simulink model "drive_impl"  (R2021a)
settings: Solver=ode23s  StartTime=0.0  StopTime=5  FixedStep=1e-4  MaxStep=1e-3  RelTol=1e-3  EnableMultiTasking=on
InitFcn:
  | run('balancing_in_one_place_code.m');
values from neighbouring files (symbols this model uses):
  Cm = Ce    (= 0.0527)    [drive_params.m]
  h_val = R*2    (= 0.228)    [drive_imp_code.m]
  J_rolik = 1/4*m_rolik*r_val^2 + 1/12*m_rolik*h_val^2    [Initial_code.m]    (also in drive_imp_code.m = 4.5350625e-08)
  J_sphere = 2*M*R^2/5    (= 0.0038988)    [Initial_code.m]    (also in drive_imp_code.m)
  K_reg = place(A,B,p)    [Initial_code.m]    (also in drive_imp_code.m)
  Kconv = Udc    [drive_params.m]
  Kfb_i = 1/In    [drive_params.m]
  Ki = Te/(2*Kfb_i*(1/Cma)*Tconv*Kconv/Cea*b)    [drive_params.m]
  Klship = 1    [drive_params.m]
  L = 0.3    [Initial_code.m]    (also in drive_imp_code.m = 0.5)
  lenght_rolik = R+r_val    (= 0.1425)    [Initial_code.m]    (also in drive_imp_code.m)
  m = 1.5    [Initial_code.m]    (also in drive_imp_code.m)
  M = 0.75    [Initial_code.m]    (also in drive_imp_code.m)
  m_rolik = 1e-5    (= 1e-05)    [Initial_code.m]    (also in drive_imp_code.m)
  R = 0.114    [Initial_code.m]    (also in drive_imp_code.m)
  r_val = R*0.25    (= 0.0285)    [Initial_code.m]    (also in drive_imp_code.m)
  T = Tk    (= 1e-05)    [drive_params.m]
  Tconv = 0.5*T    (= 5e-06)    [drive_params.m]
  Ti = Te    (= 0.000136363636364)    [drive_params.m]
  U_nom = 12    [drive_params.m]
undefined symbols (not defined in the file or in its folder): DiscIntNeverNeededParam, X, Y, Z
libraries: sm_lib x87, nesl_utility x32, fl_lib x23, simulink x10, fl_ps_legacy_lib x9, ee_lib x8, simulink_extras x4, pid_lib x1
(part 4 of 4)

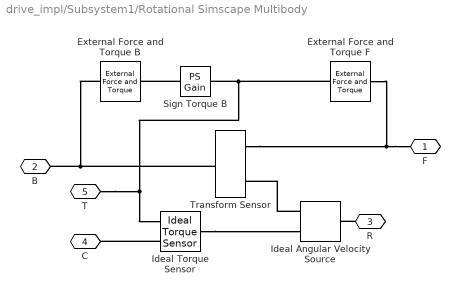
== system drive_impl/Subsystem1/Rotational Simscape Multibody ==
  External Force and Torque B : sm_lib/Forces and Torques/External Force and Torque  ForceResolutionFrame=AttachedFrame  EnableForceX=off  EnableForceY=off  EnableForceZ=off  EnableForce=off  TorqueResolutionFrame=AttachedFrame  EnableTorqueX=off  EnableTorqueY=off  EnableTorqueZ=on  EnableTorque=off
  External Force and Torque F : sm_lib/Forces and Torques/External Force and Torque  ForceResolutionFrame=AttachedFrame  EnableForceX=off  EnableForceY=off  EnableForceZ=off  EnableForce=off  TorqueResolutionFrame=AttachedFrame  EnableTorqueX=off  EnableTorqueY=off  EnableTorqueZ=on  EnableTorque=off
  Ideal Angular Velocity Source : fl_lib/Mechanical/Mechanical Sources/Ideal Angular Velocity Source
  Ideal Torque Sensor : fl_lib/Mechanical/Mechanical Sensors/Ideal Torque Sensor
  Sign Torque B : fl_ps_legacy_lib/Legacy Physical Signals/Functions/PS Gain  gain=-1
  Transform Sensor : sm_lib/Frames and Transforms/Transform Sensor  MeasurementFrame=Base  SenseAngle=off  SenseAxis=off  SenseAngle1=off  SenseAngle2=off  SenseAngle3=off  SenseQ=off  SenseR=off  SenseOmegaX=off  SenseOmegaY=off  SenseOmegaZ=on  SenseOmega1=off  SenseOmega2=off  SenseOmega3=off  SenseQDot=off  SenseRDot=off  SenseAlphaX=off  SenseAlphaY=off  SenseAlphaZ=off  SenseAlpha1=off  SenseAlpha2=off  SenseAlpha3=off  SenseQDDot=off  SenseRDDot=off  SenseX=off  SenseY=off  SenseZ=off  SenseRad=off  SenseAzim=off  SenseDist=off  SenseInc=off  SenseXDot=off  SenseYDot=off  SenseZDot=off  SenseRadDot=off  SenseAzimDot=off  SenseDistDot=off  SenseIncDot=off  SenseXDDot=off  SenseYDDot=off  SenseZDDot=off  SenseRadDDot=off  SenseAzimDDot=off  SenseDistDDot=off  SenseIncDDot=off
  F : PMIOPort  Side=Right
  B : PMIOPort  Port=2  Side=Left
  R : PMIOPort  Port=3  Side=Right
  C : PMIOPort  Port=4  Side=Left
  T : PMIOPort  Port=5  Side=Right
  connections:
  Sign Torque B/LConn1 -- T/RConn1 -- Ideal Torque Sensor/RConn2 -- External Force and Torque F/LConn1
  Sign Torque B/RConn1 -- External Force and Torque B/LConn1
  Ideal Angular Velocity Source/RConn1 -- Transform Sensor/RConn2
  F/RConn1 -- External Force and Torque F/RConn1 -- Transform Sensor/RConn1
  External Force and Torque B/RConn1 -- B/RConn1 -- Transform Sensor/LConn1
  Ideal Torque Sensor/LConn1 -- Ideal Angular Velocity Source/RConn2
  R/RConn1 -- Ideal Angular Velocity Source/LConn1
  Ideal Torque Sensor/RConn1 -- C/RConn1

== system drive_impl/Subsystem1/Subsystem1 ==
  Brick Solid : sm_lib/Body Elements/Brick Solid  GraphicAmbientColor=[0.15 0.15 0.15 1.0]  BasedOnType=Mass  BrickDimensions=[2*RolikRadius RolikLenght RolikRadius/10]  BrickDimensionUnits=m  CenterOfMass=[0 0 0]  CenterOfMassUnits=m  GraphicDiffuseColor=[1.0 0.2 0.2]  Density=1000  DensityUnits=kg/m^3  DoExposeReferenceFrame=on  GraphicEmissiveColor=[0.0 0.0 0.0 1.0]  ExportEntireGeometry=off  SerializedFrames=<Frames/>  MarkerShape=Sphere  MarkerSize=10  GraphicType=FromGeometry  InertiaType=CalculateFromGeometry  Mass=1e-6  MassUnits=kg  MomentsOfInertia=[1 1 1]  MomentsOfInertiaUnits=kg*m^2  GraphicOpacity=0.5  ProductsOfInertia=[0 0 0]  ProductsOfInertiaUnits=kg*m^2  GraphicShininess=75  GraphicSpecularColor=[0.5 0.5 0.5 1.0]  GraphicVisPropType=SimpleVisualProperties
  Brick Solid1 : sm_lib/Body Elements/Brick Solid  GraphicAmbientColor=[0.15 0.15 0.15 1.0]  BasedOnType=Mass  BrickDimensions=[2*RolikRadius RolikLenght RolikRadius/10]  BrickDimensionUnits=m  CenterOfMass=[0 0 0]  CenterOfMassUnits=m  GraphicDiffuseColor=[1.0 0.2 0.2]  Density=1000  DensityUnits=kg/m^3  DoExposeReferenceFrame=on  GraphicEmissiveColor=[0.0 0.0 0.0 1.0]  ExportEntireGeometry=off  SerializedFrames=<Frames/>  MarkerShape=Sphere  MarkerSize=10  GraphicType=FromGeometry  InertiaType=CalculateFromGeometry  Mass=1e-6  MassUnits=kg  MomentsOfInertia=[1 1 1]  MomentsOfInertiaUnits=kg*m^2  GraphicOpacity=0.5  ProductsOfInertia=[0 0 0]  ProductsOfInertiaUnits=kg*m^2  GraphicShininess=75  GraphicSpecularColor=[0.5 0.5 0.5 1.0]  GraphicVisPropType=SimpleVisualProperties
  Cylindrical Solid26 : sm_lib/Body Elements/Cylindrical Solid  GraphicAmbientColor=[0.15 0.15 0.15 1.0]  BasedOnType=Mass  CenterOfMass=[0 0 0]  CenterOfMassUnits=m  GraphicDiffuseColor=[0.2 1.0 0.2]  CylinderLength=RolikLenght  CylinderLengthUnits=m  CylinderRadius=RolikRadius  CylinderRadiusUnits=m  Density=1000  DensityUnits=kg/m^3  DoExposeReferenceFrame=on  GraphicEmissiveColor=[0.0 0.0 0.0 1.0]  ExportEntireGeometry=off  SerializedFrames=<Frames/>  MarkerShape=Sphere  MarkerSize=10  GraphicType=FromGeometry  InertiaType=CalculateFromGeometry  Mass=m_rolik  MassUnits=kg  MomentsOfInertia=[1 1 1]  MomentsOfInertiaUnits=kg*m^2  GraphicOpacity=0.6  ProductsOfInertia=[0 0 0]  ProductsOfInertiaUnits=kg*m^2  GraphicShininess=75  GraphicSpecularColor=[0.5 0.5 0.5 1.0]  GraphicVisPropType=SimpleVisualProperties
  Rigid Transform7 : sm_lib/Frames and Transforms/Rigid Transform  TranslationMethod=None  TranslationStandardOffset=0  TranslationLengthUnit=m  TranslationStandardAxis=+Z  TranslationCartesianOffset=[0 0 0]  TranslationROffset=0  TranslationROffsetUnits=m  TranslationZOffset=0  TranslationZOffsetUnits=m  TranslationThetaOffset=0  TranslationThetaOffsetUnits=deg  RotationMethod=StandardAxis  RotationAngleUnits=deg  RotationStandardAxis=+X  RotationAngle=90  RotationArbitraryAxis=[0 0 1]  FollAlignAxisA=+X  BaseAlignAxisA=+Y  FollAlignAxisB=+Y  BaseAlignAxisB=+Z  RotationSequenceAxes=FollowerAxes  RotationSequence=XYX  RotationSequenceAngles=[0 0 0]  RotationSequenceAnglesUnits=deg  RotationMatrix=[1 0 0; 0 1 0; 0 0 1]
  Rigid Transform8 : sm_lib/Frames and Transforms/Rigid Transform  TranslationMethod=None  TranslationStandardOffset=0  TranslationLengthUnit=m  TranslationStandardAxis=+Z  TranslationCartesianOffset=[0 0 0]  TranslationROffset=0  TranslationROffsetUnits=m  TranslationZOffset=0  TranslationZOffsetUnits=m  TranslationThetaOffset=0  TranslationThetaOffsetUnits=deg  RotationMethod=StandardAxis  RotationAngleUnits=deg  RotationStandardAxis=+Y  RotationAngle=90  RotationArbitraryAxis=[0 0 1]  FollAlignAxisA=+X  BaseAlignAxisA=+Y  FollAlignAxisB=+Y  BaseAlignAxisB=+Z  RotationSequenceAxes=FollowerAxes  RotationSequence=XYX  RotationSequenceAngles=[0 0 0]  RotationSequenceAnglesUnits=deg  RotationMatrix=[1 0 0; 0 1 0; 0 0 1]
  Conn1 : PMIOPort  Side=Left
  connections:
  Cylindrical Solid26/RConn1 -- Rigid Transform7/LConn1 -- Conn1/RConn1
  Brick Solid1/RConn1 -- Rigid Transform8/RConn1
  Brick Solid/RConn1 -- Rigid Transform7/RConn1 -- Rigid Transform8/LConn1

== system drive_impl/Subsystem1/Основание4 ==
  Rigid Transform : sm_lib/Frames and Transforms/Rigid Transform  TranslationMethod=None  TranslationStandardOffset=0  TranslationLengthUnit=m  TranslationStandardAxis=+Z  TranslationCartesianOffset=[0 0 0]  TranslationROffset=0  TranslationROffsetUnits=m  TranslationZOffset=0  TranslationZOffsetUnits=m  TranslationThetaOffset=0  TranslationThetaOffsetUnits=deg  RotationMethod=StandardAxis  RotationAngleUnits=deg  RotationStandardAxis=+X  RotationAngle=90  RotationArbitraryAxis=[0 0 1]  FollAlignAxisA=+X  BaseAlignAxisA=+Y  FollAlignAxisB=+Y  BaseAlignAxisB=+Z  RotationSequenceAxes=FollowerAxes  RotationSequence=XYX  RotationSequenceAngles=[0 0 0]  RotationSequenceAnglesUnits=deg  RotationMatrix=[1 0 0; 0 1 0; 0 0 1]
  Rigid Transform1 : sm_lib/Frames and Transforms/Rigid Transform  TranslationMethod=None  TranslationStandardOffset=0  TranslationLengthUnit=m  TranslationStandardAxis=+Z  TranslationCartesianOffset=[0 0 0]  TranslationROffset=0  TranslationROffsetUnits=m  TranslationZOffset=0  TranslationZOffsetUnits=m  TranslationThetaOffset=0  TranslationThetaOffsetUnits=deg  RotationMethod=StandardAxis  RotationAngleUnits=deg  RotationStandardAxis=+Y  RotationAngle=90  RotationArbitraryAxis=[0 0 1]  FollAlignAxisA=+X  BaseAlignAxisA=+Y  FollAlignAxisB=+Y  BaseAlignAxisB=+Z  RotationSequenceAxes=FollowerAxes  RotationSequence=XYX  RotationSequenceAngles=[0 0 0]  RotationSequenceAnglesUnits=deg  RotationMatrix=[1 0 0; 0 1 0; 0 0 1]
  Solid1 : sm_lib/Body Elements/Spherical Solid  GraphicAmbientColor=[0.15 0.15 0.15 1.0]  BasedOnType=Mass  CenterOfMass=[0 0 0]  CenterOfMassUnits=m  GraphicDiffuseColor=[1.0 1.0 0.0]  Density=1000  DensityUnits=kg/m^3  DoExposeReferenceFrame=on  GraphicEmissiveColor=[0.0 0.0 0.0 1.0]  ExportEntireGeometry=off  SerializedExposedGeometries=<ExposedGeometries/>  SerializedFrames=<Frames/>  MarkerShape=Sphere  MarkerSize=10  GraphicType=FromGeometry  InertiaType=CalculateFromGeometry  Mass=Mass  MassUnits=kg  MomentsOfInertia=[1 1 1]  MomentsOfInertiaUnits=kg*m^2  GraphicOpacity=1.0  ProductsOfInertia=[1 1 1]  ProductsOfInertiaUnits=kg*m^2  GraphicShininess=75  GraphicSpecularColor=[0.5 0.5 0.5 1.0]  SphereRadius=SphereRadius  SphereRadiusUnits=m  GraphicVisPropType=SimpleVisualProperties
  Solid2 : sm_lib/Body Elements/Revolved Solid  GraphicAmbientColor=[0.15 0.15 0.15 1.0]  BasedOnType=Mass  CenterOfMass=[0 0 0]  CenterOfMassUnits=m  GraphicDiffuseColor=[1.0 0.0 0.0]  ExportConvexHullGeometry=off  Density=1000  DensityUnits=kg/m^3  DoExposeReferenceFrame=on  GraphicEmissiveColor=[0.0 0.0 0.0 1.0]  ExportEntireGeometry=off  SerializedFrames=<Frames/>  MarkerShape=Sphere  MarkerSize=10  GraphicType=FromGeometry  InertiaType=CalculateFromGeometry  Mass=0  MassUnits=kg  MomentsOfInertia=[1 1 1]  MomentsOfInertiaUnits=kg*m^2  GraphicOpacity=0.5  ProductsOfInertia=[1 1 1]  ProductsOfInertiaUnits=kg*m^2  RevolutionCrossSection=[0 SphereRadius*perc1; 0 -SphereRadius*perc1; SphereRadius*1.01 -SphereRadius*perc1; SphereRadius*1.01 SphereRadius*perc1]  RevolutionCrossSectionUnits=m  RevolutionAngle=180  RevolutionAngleUnits=deg  RevolutionExtent=Full  GraphicShininess=75  GraphicSpecularColor=[0.5 0.5 0.5 1.0]  GraphicVisPropType=SimpleVisualProperties
  Solid3 : sm_lib/Body Elements/Revolved Solid  GraphicAmbientColor=[0.15 0.15 0.15 1.0]  BasedOnType=Mass  CenterOfMass=[0 0 0]  CenterOfMassUnits=m  GraphicDiffuseColor=[1.0 0.0 0.0]  ExportConvexHullGeometry=off  Density=1000  DensityUnits=kg/m^3  DoExposeReferenceFrame=on  GraphicEmissiveColor=[0.0 0.0 0.0 1.0]  ExportEntireGeometry=off  SerializedFrames=<Frames/>  MarkerShape=Sphere  MarkerSize=10  GraphicType=FromGeometry  InertiaType=CalculateFromGeometry  Mass=0  MassUnits=kg  MomentsOfInertia=[1 1 1]  MomentsOfInertiaUnits=kg*m^2  GraphicOpacity=0.5  ProductsOfInertia=[1 1 1]  ProductsOfInertiaUnits=kg*m^2  RevolutionCrossSection=[0 SphereRadius*perc1; 0 -SphereRadius*perc1; SphereRadius*perc2 -SphereRadius*perc1; SphereRadius*perc2 SphereRadius*perc1]  RevolutionCrossSectionUnits=m  RevolutionAngle=180  RevolutionAngleUnits=deg  RevolutionExtent=Full  GraphicShininess=75  GraphicSpecularColor=[0.5 0.5 0.5 1.0]  GraphicVisPropType=SimpleVisualProperties
  Solid4 : sm_lib/Body Elements/Revolved Solid  GraphicAmbientColor=[0.15 0.15 0.15 1.0]  BasedOnType=Mass  CenterOfMass=[0 0 0]  CenterOfMassUnits=m  GraphicDiffuseColor=[1.0 0.0 0.0]  ExportConvexHullGeometry=off  Density=1000  DensityUnits=kg/m^3  DoExposeReferenceFrame=on  GraphicEmissiveColor=[0.0 0.0 0.0 1.0]  ExportEntireGeometry=off  SerializedFrames=<Frames/>  MarkerShape=Sphere  MarkerSize=10  GraphicType=FromGeometry  InertiaType=CalculateFromGeometry  Mass=0  MassUnits=kg  MomentsOfInertia=[1 1 1]  MomentsOfInertiaUnits=kg*m^2  GraphicOpacity=0.5  ProductsOfInertia=[1 1 1]  ProductsOfInertiaUnits=kg*m^2  RevolutionCrossSection=[0 SphereRadius*perc1; 0 -SphereRadius*perc1; SphereRadius*perc2 -SphereRadius*perc1; SphereRadius*perc2 SphereRadius*perc1]  RevolutionCrossSectionUnits=m  RevolutionAngle=180  RevolutionAngleUnits=deg  RevolutionExtent=Full  GraphicShininess=75  GraphicSpecularColor=[0.5 0.5 0.5 1.0]  GraphicVisPropType=SimpleVisualProperties
  Conn1 : PMIOPort  Side=Left
  connections:
  Rigid Transform/LConn1 -- Solid2/RConn1 -- Solid1/RConn1 -- Conn1/RConn1
  Solid4/RConn1 -- Rigid Transform1/RConn1
  Rigid Transform1/LConn1 -- Rigid Transform/RConn1 -- Solid3/RConn1

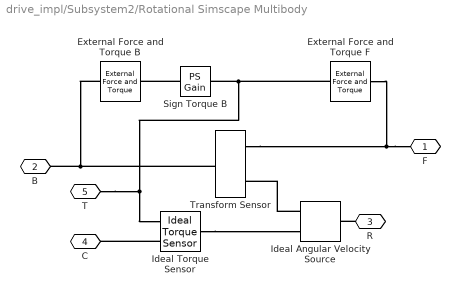
== system drive_impl/Subsystem2/Rotational Simscape Multibody ==
  External Force and Torque B : sm_lib/Forces and Torques/External Force and Torque  ForceResolutionFrame=AttachedFrame  EnableForceX=off  EnableForceY=off  EnableForceZ=off  EnableForce=off  TorqueResolutionFrame=AttachedFrame  EnableTorqueX=off  EnableTorqueY=off  EnableTorqueZ=on  EnableTorque=off
  External Force and Torque F : sm_lib/Forces and Torques/External Force and Torque  ForceResolutionFrame=AttachedFrame  EnableForceX=off  EnableForceY=off  EnableForceZ=off  EnableForce=off  TorqueResolutionFrame=AttachedFrame  EnableTorqueX=off  EnableTorqueY=off  EnableTorqueZ=on  EnableTorque=off
  Ideal Angular Velocity Source : fl_lib/Mechanical/Mechanical Sources/Ideal Angular Velocity Source
  Ideal Torque Sensor : fl_lib/Mechanical/Mechanical Sensors/Ideal Torque Sensor
  Sign Torque B : fl_ps_legacy_lib/Legacy Physical Signals/Functions/PS Gain  gain=-1
  Transform Sensor : sm_lib/Frames and Transforms/Transform Sensor  MeasurementFrame=Base  SenseAngle=off  SenseAxis=off  SenseAngle1=off  SenseAngle2=off  SenseAngle3=off  SenseQ=off  SenseR=off  SenseOmegaX=off  SenseOmegaY=off  SenseOmegaZ=on  SenseOmega1=off  SenseOmega2=off  SenseOmega3=off  SenseQDot=off  SenseRDot=off  SenseAlphaX=off  SenseAlphaY=off  SenseAlphaZ=off  SenseAlpha1=off  SenseAlpha2=off  SenseAlpha3=off  SenseQDDot=off  SenseRDDot=off  SenseX=off  SenseY=off  SenseZ=off  SenseRad=off  SenseAzim=off  SenseDist=off  SenseInc=off  SenseXDot=off  SenseYDot=off  SenseZDot=off  SenseRadDot=off  SenseAzimDot=off  SenseDistDot=off  SenseIncDot=off  SenseXDDot=off  SenseYDDot=off  SenseZDDot=off  SenseRadDDot=off  SenseAzimDDot=off  SenseDistDDot=off  SenseIncDDot=off
  F : PMIOPort  Side=Right
  B : PMIOPort  Port=2  Side=Left
  R : PMIOPort  Port=3  Side=Right
  C : PMIOPort  Port=4  Side=Left
  T : PMIOPort  Port=5  Side=Right
  connections:
  Sign Torque B/LConn1 -- T/RConn1 -- Ideal Torque Sensor/RConn2 -- External Force and Torque F/LConn1
  Sign Torque B/RConn1 -- External Force and Torque B/LConn1
  Ideal Angular Velocity Source/RConn1 -- Transform Sensor/RConn2
  F/RConn1 -- External Force and Torque F/RConn1 -- Transform Sensor/RConn1
  External Force and Torque B/RConn1 -- B/RConn1 -- Transform Sensor/LConn1
  Ideal Torque Sensor/LConn1 -- Ideal Angular Velocity Source/RConn2
  R/RConn1 -- Ideal Angular Velocity Source/LConn1
  Ideal Torque Sensor/RConn1 -- C/RConn1

== system drive_impl/Subsystem2/Основание4 ==
  Rigid Transform : sm_lib/Frames and Transforms/Rigid Transform  TranslationMethod=None  TranslationStandardOffset=0  TranslationLengthUnit=m  TranslationStandardAxis=+Z  TranslationCartesianOffset=[0 0 0]  TranslationROffset=0  TranslationROffsetUnits=m  TranslationZOffset=0  TranslationZOffsetUnits=m  TranslationThetaOffset=0  TranslationThetaOffsetUnits=deg  RotationMethod=StandardAxis  RotationAngleUnits=deg  RotationStandardAxis=+X  RotationAngle=90  RotationArbitraryAxis=[0 0 1]  FollAlignAxisA=+X  BaseAlignAxisA=+Y  FollAlignAxisB=+Y  BaseAlignAxisB=+Z  RotationSequenceAxes=FollowerAxes  RotationSequence=XYX  RotationSequenceAngles=[0 0 0]  RotationSequenceAnglesUnits=deg  RotationMatrix=[1 0 0; 0 1 0; 0 0 1]
  Rigid Transform1 : sm_lib/Frames and Transforms/Rigid Transform  TranslationMethod=None  TranslationStandardOffset=0  TranslationLengthUnit=m  TranslationStandardAxis=+Z  TranslationCartesianOffset=[0 0 0]  TranslationROffset=0  TranslationROffsetUnits=m  TranslationZOffset=0  TranslationZOffsetUnits=m  TranslationThetaOffset=0  TranslationThetaOffsetUnits=deg  RotationMethod=StandardAxis  RotationAngleUnits=deg  RotationStandardAxis=+Y  RotationAngle=90  RotationArbitraryAxis=[0 0 1]  FollAlignAxisA=+X  BaseAlignAxisA=+Y  FollAlignAxisB=+Y  BaseAlignAxisB=+Z  RotationSequenceAxes=FollowerAxes  RotationSequence=XYX  RotationSequenceAngles=[0 0 0]  RotationSequenceAnglesUnits=deg  RotationMatrix=[1 0 0; 0 1 0; 0 0 1]
  Solid1 : sm_lib/Body Elements/Spherical Solid  GraphicAmbientColor=[0.15 0.15 0.15 1.0]  BasedOnType=Mass  CenterOfMass=[0 0 0]  CenterOfMassUnits=m  GraphicDiffuseColor=[1.0 1.0 0.0]  Density=1000  DensityUnits=kg/m^3  DoExposeReferenceFrame=on  GraphicEmissiveColor=[0.0 0.0 0.0 1.0]  ExportEntireGeometry=off  SerializedExposedGeometries=<ExposedGeometries/>  SerializedFrames=<Frames/>  MarkerShape=Sphere  MarkerSize=10  GraphicType=FromGeometry  InertiaType=CalculateFromGeometry  Mass=Mass  MassUnits=kg  MomentsOfInertia=[1 1 1]  MomentsOfInertiaUnits=kg*m^2  GraphicOpacity=1.0  ProductsOfInertia=[1 1 1]  ProductsOfInertiaUnits=kg*m^2  GraphicShininess=75  GraphicSpecularColor=[0.5 0.5 0.5 1.0]  SphereRadius=SphereRadius  SphereRadiusUnits=m  GraphicVisPropType=SimpleVisualProperties
  Solid2 : sm_lib/Body Elements/Revolved Solid  GraphicAmbientColor=[0.15 0.15 0.15 1.0]  BasedOnType=Mass  CenterOfMass=[0 0 0]  CenterOfMassUnits=m  GraphicDiffuseColor=[1.0 0.0 0.0]  ExportConvexHullGeometry=off  Density=1000  DensityUnits=kg/m^3  DoExposeReferenceFrame=on  GraphicEmissiveColor=[0.0 0.0 0.0 1.0]  ExportEntireGeometry=off  SerializedFrames=<Frames/>  MarkerShape=Sphere  MarkerSize=10  GraphicType=FromGeometry  InertiaType=CalculateFromGeometry  Mass=0  MassUnits=kg  MomentsOfInertia=[1 1 1]  MomentsOfInertiaUnits=kg*m^2  GraphicOpacity=0.5  ProductsOfInertia=[1 1 1]  ProductsOfInertiaUnits=kg*m^2  RevolutionCrossSection=[0 SphereRadius*perc1; 0 -SphereRadius*perc1; SphereRadius*1.01 -SphereRadius*perc1; SphereRadius*1.01 SphereRadius*perc1]  RevolutionCrossSectionUnits=m  RevolutionAngle=180  RevolutionAngleUnits=deg  RevolutionExtent=Full  GraphicShininess=75  GraphicSpecularColor=[0.5 0.5 0.5 1.0]  GraphicVisPropType=SimpleVisualProperties
  Solid3 : sm_lib/Body Elements/Revolved Solid  GraphicAmbientColor=[0.15 0.15 0.15 1.0]  BasedOnType=Mass  CenterOfMass=[0 0 0]  CenterOfMassUnits=m  GraphicDiffuseColor=[1.0 0.0 0.0]  ExportConvexHullGeometry=off  Density=1000  DensityUnits=kg/m^3  DoExposeReferenceFrame=on  GraphicEmissiveColor=[0.0 0.0 0.0 1.0]  ExportEntireGeometry=off  SerializedFrames=<Frames/>  MarkerShape=Sphere  MarkerSize=10  GraphicType=FromGeometry  InertiaType=CalculateFromGeometry  Mass=0  MassUnits=kg  MomentsOfInertia=[1 1 1]  MomentsOfInertiaUnits=kg*m^2  GraphicOpacity=0.5  ProductsOfInertia=[1 1 1]  ProductsOfInertiaUnits=kg*m^2  RevolutionCrossSection=[0 SphereRadius*perc1; 0 -SphereRadius*perc1; SphereRadius*perc2 -SphereRadius*perc1; SphereRadius*perc2 SphereRadius*perc1]  RevolutionCrossSectionUnits=m  RevolutionAngle=180  RevolutionAngleUnits=deg  RevolutionExtent=Full  GraphicShininess=75  GraphicSpecularColor=[0.5 0.5 0.5 1.0]  GraphicVisPropType=SimpleVisualProperties
  Solid4 : sm_lib/Body Elements/Revolved Solid  GraphicAmbientColor=[0.15 0.15 0.15 1.0]  BasedOnType=Mass  CenterOfMass=[0 0 0]  CenterOfMassUnits=m  GraphicDiffuseColor=[1.0 0.0 0.0]  ExportConvexHullGeometry=off  Density=1000  DensityUnits=kg/m^3  DoExposeReferenceFrame=on  GraphicEmissiveColor=[0.0 0.0 0.0 1.0]  ExportEntireGeometry=off  SerializedFrames=<Frames/>  MarkerShape=Sphere  MarkerSize=10  GraphicType=FromGeometry  InertiaType=CalculateFromGeometry  Mass=0  MassUnits=kg  MomentsOfInertia=[1 1 1]  MomentsOfInertiaUnits=kg*m^2  GraphicOpacity=0.5  ProductsOfInertia=[1 1 1]  ProductsOfInertiaUnits=kg*m^2  RevolutionCrossSection=[0 SphereRadius*perc1; 0 -SphereRadius*perc1; SphereRadius*perc2 -SphereRadius*perc1; SphereRadius*perc2 SphereRadius*perc1]  RevolutionCrossSectionUnits=m  RevolutionAngle=180  RevolutionAngleUnits=deg  RevolutionExtent=Full  GraphicShininess=75  GraphicSpecularColor=[0.5 0.5 0.5 1.0]  GraphicVisPropType=SimpleVisualProperties
  Conn1 : PMIOPort  Side=Left
  connections:
  Rigid Transform/LConn1 -- Solid2/RConn1 -- Solid1/RConn1 -- Conn1/RConn1
  Solid4/RConn1 -- Rigid Transform1/RConn1
  Rigid Transform1/LConn1 -- Rigid Transform/RConn1 -- Solid3/RConn1

== system drive_impl/Subsystem3/DC Current Sensor ==
  Current Sensor : fl_lib/Electrical/Electrical Sensors/Current Sensor
      settings: LogSimulationData=on
  PS-Simulink Converter : nesl_utility/PS-Simulink Converter  PhysicalDomain=network_engine_domain  SubClassName=ps_output  LeftPortType=input  RightPortType=output  PseudoPeriodic=off  Frequencies=[]  Unit=1  AffineConversion=off
      settings: SourceProductBaseCode=PW,SS
  - : PMIOPort  Side=Left
  + : PMIOPort  Port=2  Side=Right
  tag scope: i_dc=global
  wires:
  PS-Simulink Converter/1 -> [i_dc]
  connections:
  Current Sensor/RConn2 -- -/RConn1
  +/RConn1 -- Current Sensor/LConn1
  Current Sensor/RConn1 -- PS-Simulink Converter/LConn1

== system drive_impl/Subsystem3/DC Voltage Sensor ==
  PS-Simulink Converter : nesl_utility/PS-Simulink Converter  PhysicalDomain=network_engine_domain  SubClassName=ps_output  LeftPortType=input  RightPortType=output  PseudoPeriodic=off  Frequencies=[]  Unit=1  AffineConversion=off
      settings: SourceProductBaseCode=PW,SS
  Voltage Sensor : fl_lib/Electrical/Electrical Sensors/Voltage Sensor
      settings: LogSimulationData=on
  - : PMIOPort  Side=Left
  + : PMIOPort  Port=2  Side=Right
  tag scope: v_dc=global
  wires:
  PS-Simulink Converter/1 -> [v_dc]
  connections:
  Voltage Sensor/LConn1 -- +/RConn1
  Voltage Sensor/RConn1 -- PS-Simulink Converter/LConn1
  Voltage Sensor/RConn2 -- -/RConn1

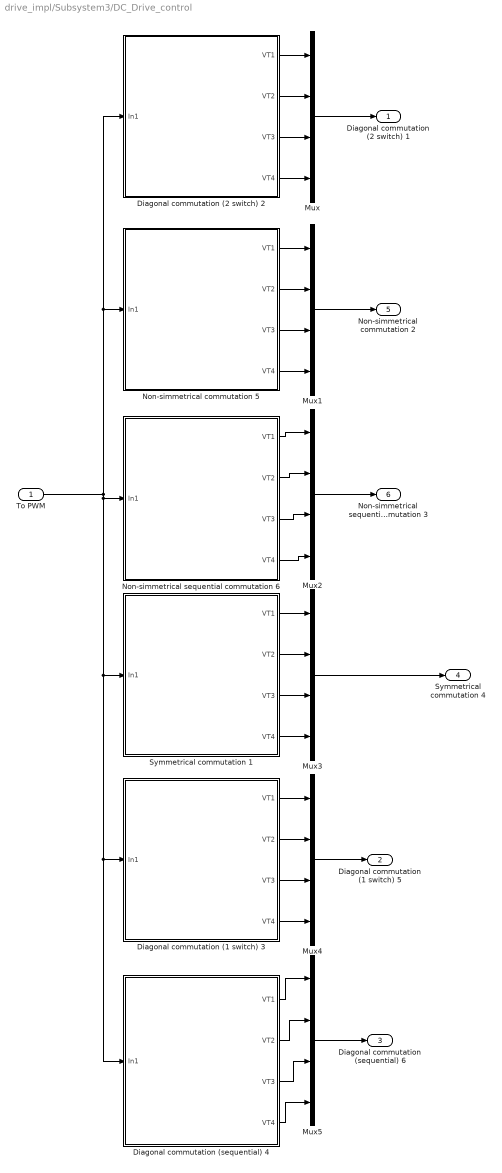
== system drive_impl/Subsystem3/DC_Drive_control ==
  To PWM : Inport
  Diagonal commutation (1 switch) 3 : Subsystem
  Diagonal commutation (2 switch) 2 : Subsystem
  Diagonal commutation (sequential) 4 : Subsystem
  Mux{,1..5} (6 alike) : Mux
  Non-simmetrical commutation 5 : Subsystem
  "Non-simmetrical sequential commutation 6 " : Subsystem
  Symmetrical commutation 1 : Subsystem
  Diagonal commutation (2 switch) 1 : Outport  VectorParamsAs1DForOutWhenUnconnected=off
  Diagonal commutation (1 switch) 5 : Outport  Port=2  VectorParamsAs1DForOutWhenUnconnected=off
  Diagonal commutation (sequential) 6 : Outport  Port=3  VectorParamsAs1DForOutWhenUnconnected=off
  Symmetrical commutation 4 : Outport  Port=4  VectorParamsAs1DForOutWhenUnconnected=off
  Non-simmetrical commutation 2 : Outport  Port=5  VectorParamsAs1DForOutWhenUnconnected=off
  "Non-simmetrical sequential commutation 3 " : Outport  Port=6  VectorParamsAs1DForOutWhenUnconnected=off
  wires:
  To PWM/1 -> "Non-simmetrical sequential commutation 6 "/1(In1), Diagonal commutation (1 switch) 3/1(In1), Diagonal commutation (sequential) 4/1(In1), Symmetrical commutation 1/1(In1), Diagonal commutation (2 switch) 2/1(In1), Non-simmetrical commutation 5/1(In1)
  Diagonal commutation (2 switch) 2/1(VT1) -> Mux/1
  Diagonal commutation (2 switch) 2/2(VT2) -> Mux/2
  Diagonal commutation (2 switch) 2/3(VT3) -> Mux/3
  Diagonal commutation (2 switch) 2/4(VT4) -> Mux/4
  Non-simmetrical commutation 5/1(VT1) -> Mux1/1
  Non-simmetrical commutation 5/2(VT2) -> Mux1/2
  Non-simmetrical commutation 5/3(VT3) -> Mux1/3
  Non-simmetrical commutation 5/4(VT4) -> Mux1/4
  "Non-simmetrical sequential commutation 6 "/3(VT3) -> Mux2/3
  "Non-simmetrical sequential commutation 6 "/4(VT4) -> Mux2/4
  "Non-simmetrical sequential commutation 6 "/2(VT2) -> Mux2/2
  Symmetrical commutation 1/4(VT4) -> Mux3/4
  Symmetrical commutation 1/1(VT1) -> Mux3/1
  "Non-simmetrical sequential commutation 6 "/1(VT1) -> Mux2/1
  Symmetrical commutation 1/3(VT3) -> Mux3/3
  Symmetrical commutation 1/2(VT2) -> Mux3/2
  Diagonal commutation (1 switch) 3/3(VT3) -> Mux4/3
  Diagonal commutation (1 switch) 3/4(VT4) -> Mux4/4
  Diagonal commutation (1 switch) 3/2(VT2) -> Mux4/2
  Diagonal commutation (sequential) 4/4(VT4) -> Mux5/4
  Diagonal commutation (sequential) 4/1(VT1) -> Mux5/1
  Diagonal commutation (1 switch) 3/1(VT1) -> Mux4/1
  Mux3/1 -> Symmetrical commutation 4/1
  Mux/1 -> Diagonal commutation (2 switch) 1/1
  Mux4/1 -> Diagonal commutation (1 switch) 5/1
  Mux5/1 -> Diagonal commutation (sequential) 6/1
  Mux1/1 -> Non-simmetrical commutation 2/1
  Mux2/1 -> "Non-simmetrical sequential commutation 3 "/1
  Diagonal commutation (sequential) 4/2(VT2) -> Mux5/2
  Diagonal commutation (sequential) 4/3(VT3) -> Mux5/3

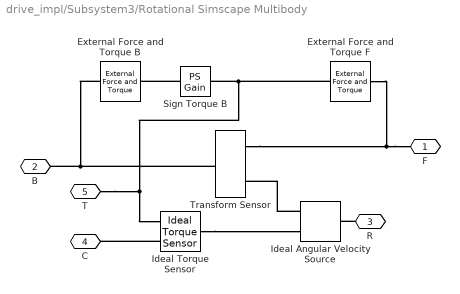
== system drive_impl/Subsystem3/Rotational Simscape Multibody ==
  External Force and Torque B : sm_lib/Forces and Torques/External Force and Torque  ForceResolutionFrame=AttachedFrame  EnableForceX=off  EnableForceY=off  EnableForceZ=off  EnableForce=off  TorqueResolutionFrame=AttachedFrame  EnableTorqueX=off  EnableTorqueY=off  EnableTorqueZ=on  EnableTorque=off
  External Force and Torque F : sm_lib/Forces and Torques/External Force and Torque  ForceResolutionFrame=AttachedFrame  EnableForceX=off  EnableForceY=off  EnableForceZ=off  EnableForce=off  TorqueResolutionFrame=AttachedFrame  EnableTorqueX=off  EnableTorqueY=off  EnableTorqueZ=on  EnableTorque=off
  Ideal Angular Velocity Source : fl_lib/Mechanical/Mechanical Sources/Ideal Angular Velocity Source
  Ideal Torque Sensor : fl_lib/Mechanical/Mechanical Sensors/Ideal Torque Sensor
  Sign Torque B : fl_ps_legacy_lib/Legacy Physical Signals/Functions/PS Gain  gain=-1
  Transform Sensor : sm_lib/Frames and Transforms/Transform Sensor  MeasurementFrame=Base  SenseAngle=off  SenseAxis=off  SenseAngle1=off  SenseAngle2=off  SenseAngle3=off  SenseQ=off  SenseR=off  SenseOmegaX=off  SenseOmegaY=off  SenseOmegaZ=on  SenseOmega1=off  SenseOmega2=off  SenseOmega3=off  SenseQDot=off  SenseRDot=off  SenseAlphaX=off  SenseAlphaY=off  SenseAlphaZ=off  SenseAlpha1=off  SenseAlpha2=off  SenseAlpha3=off  SenseQDDot=off  SenseRDDot=off  SenseX=off  SenseY=off  SenseZ=off  SenseRad=off  SenseAzim=off  SenseDist=off  SenseInc=off  SenseXDot=off  SenseYDot=off  SenseZDot=off  SenseRadDot=off  SenseAzimDot=off  SenseDistDot=off  SenseIncDot=off  SenseXDDot=off  SenseYDDot=off  SenseZDDot=off  SenseRadDDot=off  SenseAzimDDot=off  SenseDistDDot=off  SenseIncDDot=off
  F : PMIOPort  Side=Right
  B : PMIOPort  Port=2  Side=Left
  R : PMIOPort  Port=3  Side=Right
  C : PMIOPort  Port=4  Side=Left
  T : PMIOPort  Port=5  Side=Right
  connections:
  Sign Torque B/LConn1 -- T/RConn1 -- Ideal Torque Sensor/RConn2 -- External Force and Torque F/LConn1
  Sign Torque B/RConn1 -- External Force and Torque B/LConn1
  Ideal Angular Velocity Source/RConn1 -- Transform Sensor/RConn2
  F/RConn1 -- External Force and Torque F/RConn1 -- Transform Sensor/RConn1
  External Force and Torque B/RConn1 -- B/RConn1 -- Transform Sensor/LConn1
  Ideal Torque Sensor/LConn1 -- Ideal Angular Velocity Source/RConn2
  R/RConn1 -- Ideal Angular Velocity Source/LConn1
  Ideal Torque Sensor/RConn1 -- C/RConn1

== system drive_impl/Subsystem3/Основание4 ==
  Rigid Transform : sm_lib/Frames and Transforms/Rigid Transform  TranslationMethod=None  TranslationStandardOffset=0  TranslationLengthUnit=m  TranslationStandardAxis=+Z  TranslationCartesianOffset=[0 0 0]  TranslationROffset=0  TranslationROffsetUnits=m  TranslationZOffset=0  TranslationZOffsetUnits=m  TranslationThetaOffset=0  TranslationThetaOffsetUnits=deg  RotationMethod=StandardAxis  RotationAngleUnits=deg  RotationStandardAxis=+X  RotationAngle=90  RotationArbitraryAxis=[0 0 1]  FollAlignAxisA=+X  BaseAlignAxisA=+Y  FollAlignAxisB=+Y  BaseAlignAxisB=+Z  RotationSequenceAxes=FollowerAxes  RotationSequence=XYX  RotationSequenceAngles=[0 0 0]  RotationSequenceAnglesUnits=deg  RotationMatrix=[1 0 0; 0 1 0; 0 0 1]
  Rigid Transform1 : sm_lib/Frames and Transforms/Rigid Transform  TranslationMethod=None  TranslationStandardOffset=0  TranslationLengthUnit=m  TranslationStandardAxis=+Z  TranslationCartesianOffset=[0 0 0]  TranslationROffset=0  TranslationROffsetUnits=m  TranslationZOffset=0  TranslationZOffsetUnits=m  TranslationThetaOffset=0  TranslationThetaOffsetUnits=deg  RotationMethod=StandardAxis  RotationAngleUnits=deg  RotationStandardAxis=+Y  RotationAngle=90  RotationArbitraryAxis=[0 0 1]  FollAlignAxisA=+X  BaseAlignAxisA=+Y  FollAlignAxisB=+Y  BaseAlignAxisB=+Z  RotationSequenceAxes=FollowerAxes  RotationSequence=XYX  RotationSequenceAngles=[0 0 0]  RotationSequenceAnglesUnits=deg  RotationMatrix=[1 0 0; 0 1 0; 0 0 1]
  Solid1 : sm_lib/Body Elements/Spherical Solid  GraphicAmbientColor=[0.15 0.15 0.15 1.0]  BasedOnType=Mass  CenterOfMass=[0 0 0]  CenterOfMassUnits=m  GraphicDiffuseColor=[1.0 1.0 0.0]  Density=1000  DensityUnits=kg/m^3  DoExposeReferenceFrame=on  GraphicEmissiveColor=[0.0 0.0 0.0 1.0]  ExportEntireGeometry=off  SerializedExposedGeometries=<ExposedGeometries/>  SerializedFrames=<Frames/>  MarkerShape=Sphere  MarkerSize=10  GraphicType=FromGeometry  InertiaType=CalculateFromGeometry  Mass=Mass  MassUnits=kg  MomentsOfInertia=[1 1 1]  MomentsOfInertiaUnits=kg*m^2  GraphicOpacity=1.0  ProductsOfInertia=[1 1 1]  ProductsOfInertiaUnits=kg*m^2  GraphicShininess=75  GraphicSpecularColor=[0.5 0.5 0.5 1.0]  SphereRadius=SphereRadius  SphereRadiusUnits=m  GraphicVisPropType=SimpleVisualProperties
  Solid2 : sm_lib/Body Elements/Revolved Solid  GraphicAmbientColor=[0.15 0.15 0.15 1.0]  BasedOnType=Mass  CenterOfMass=[0 0 0]  CenterOfMassUnits=m  GraphicDiffuseColor=[1.0 0.0 0.0]  ExportConvexHullGeometry=off  Density=1000  DensityUnits=kg/m^3  DoExposeReferenceFrame=on  GraphicEmissiveColor=[0.0 0.0 0.0 1.0]  ExportEntireGeometry=off  SerializedFrames=<Frames/>  MarkerShape=Sphere  MarkerSize=10  GraphicType=FromGeometry  InertiaType=CalculateFromGeometry  Mass=0  MassUnits=kg  MomentsOfInertia=[1 1 1]  MomentsOfInertiaUnits=kg*m^2  GraphicOpacity=0.5  ProductsOfInertia=[1 1 1]  ProductsOfInertiaUnits=kg*m^2  RevolutionCrossSection=[0 SphereRadius*perc1; 0 -SphereRadius*perc1; SphereRadius*1.01 -SphereRadius*perc1; SphereRadius*1.01 SphereRadius*perc1]  RevolutionCrossSectionUnits=m  RevolutionAngle=180  RevolutionAngleUnits=deg  RevolutionExtent=Full  GraphicShininess=75  GraphicSpecularColor=[0.5 0.5 0.5 1.0]  GraphicVisPropType=SimpleVisualProperties
  Solid3 : sm_lib/Body Elements/Revolved Solid  GraphicAmbientColor=[0.15 0.15 0.15 1.0]  BasedOnType=Mass  CenterOfMass=[0 0 0]  CenterOfMassUnits=m  GraphicDiffuseColor=[1.0 0.0 0.0]  ExportConvexHullGeometry=off  Density=1000  DensityUnits=kg/m^3  DoExposeReferenceFrame=on  GraphicEmissiveColor=[0.0 0.0 0.0 1.0]  ExportEntireGeometry=off  SerializedFrames=<Frames/>  MarkerShape=Sphere  MarkerSize=10  GraphicType=FromGeometry  InertiaType=CalculateFromGeometry  Mass=0  MassUnits=kg  MomentsOfInertia=[1 1 1]  MomentsOfInertiaUnits=kg*m^2  GraphicOpacity=0.5  ProductsOfInertia=[1 1 1]  ProductsOfInertiaUnits=kg*m^2  RevolutionCrossSection=[0 SphereRadius*perc1; 0 -SphereRadius*perc1; SphereRadius*perc2 -SphereRadius*perc1; SphereRadius*perc2 SphereRadius*perc1]  RevolutionCrossSectionUnits=m  RevolutionAngle=180  RevolutionAngleUnits=deg  RevolutionExtent=Full  GraphicShininess=75  GraphicSpecularColor=[0.5 0.5 0.5 1.0]  GraphicVisPropType=SimpleVisualProperties
  Solid4 : sm_lib/Body Elements/Revolved Solid  GraphicAmbientColor=[0.15 0.15 0.15 1.0]  BasedOnType=Mass  CenterOfMass=[0 0 0]  CenterOfMassUnits=m  GraphicDiffuseColor=[1.0 0.0 0.0]  ExportConvexHullGeometry=off  Density=1000  DensityUnits=kg/m^3  DoExposeReferenceFrame=on  GraphicEmissiveColor=[0.0 0.0 0.0 1.0]  ExportEntireGeometry=off  SerializedFrames=<Frames/>  MarkerShape=Sphere  MarkerSize=10  GraphicType=FromGeometry  InertiaType=CalculateFromGeometry  Mass=0  MassUnits=kg  MomentsOfInertia=[1 1 1]  MomentsOfInertiaUnits=kg*m^2  GraphicOpacity=0.5  ProductsOfInertia=[1 1 1]  ProductsOfInertiaUnits=kg*m^2  RevolutionCrossSection=[0 SphereRadius*perc1; 0 -SphereRadius*perc1; SphereRadius*perc2 -SphereRadius*perc1; SphereRadius*perc2 SphereRadius*perc1]  RevolutionCrossSectionUnits=m  RevolutionAngle=180  RevolutionAngleUnits=deg  RevolutionExtent=Full  GraphicShininess=75  GraphicSpecularColor=[0.5 0.5 0.5 1.0]  GraphicVisPropType=SimpleVisualProperties
  Conn1 : PMIOPort  Side=Left
  connections:
  Rigid Transform/LConn1 -- Solid2/RConn1 -- Solid1/RConn1 -- Conn1/RConn1
  Solid4/RConn1 -- Rigid Transform1/RConn1
  Rigid Transform1/LConn1 -- Rigid Transform/RConn1 -- Solid3/RConn1

== system drive_impl/Subsystem3/DC_Drive_control/Diagonal commutation (1 switch) 3 ==
  In1 : Inport
  Compare To Zero1 : simulink/Logic and Bit Operations/Compare To Zero  relop=<  OutDataTypeStr=boolean
  Compare To Zero2 : simulink/Logic and Bit Operations/Compare To Zero  relop=>  OutDataTypeStr=boolean
  Relational Operator : RelationalOperator  Operator=>  OutDataTypeStr=boolean  RndMeth=Nearest
  Repeating Sequence : simulink/Sources/Repeating Sequence  rep_seq_t="[0  T ]"  rep_seq_y=[1 0]
  VT1 : Outport  VectorParamsAs1DForOutWhenUnconnected=off
  VT2 : Outport  Port=2  VectorParamsAs1DForOutWhenUnconnected=off
  VT3 : Outport  Port=3  VectorParamsAs1DForOutWhenUnconnected=off
  VT4 : Outport  Port=4  VectorParamsAs1DForOutWhenUnconnected=off
  wires:
  Compare To Zero2/1 -> VT4/1
  Compare To Zero1/1 -> VT3/1, VT2/1
  In1/1 -> Relational Operator/1
  Repeating Sequence/1 -> Relational Operator/2, Compare To Zero1/1, Compare To Zero2/1
  Relational Operator/1 -> VT1/1

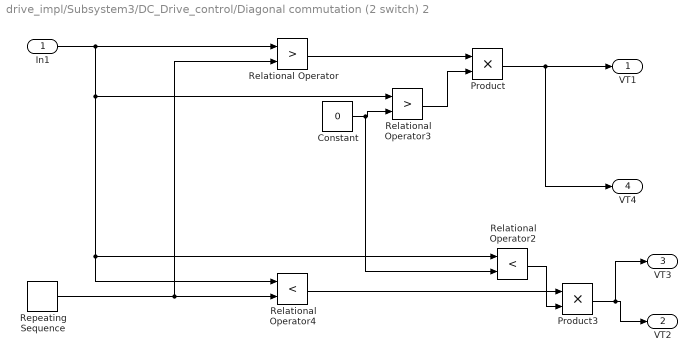
== system drive_impl/Subsystem3/DC_Drive_control/Diagonal commutation (2 switch) 2 ==
  In1 : Inport
  Constant : Constant  Value=0
  Product : Product
  Product3 : Product
  Relational Operator : RelationalOperator  Operator=>  OutDataTypeStr=boolean  RndMeth=Nearest
  Relational Operator2 : RelationalOperator  Operator=<  OutDataTypeStr=boolean  RndMeth=Nearest
  Relational Operator3 : RelationalOperator  Operator=>  OutDataTypeStr=boolean  RndMeth=Nearest
  Relational Operator4 : RelationalOperator  Operator=<  OutDataTypeStr=boolean  RndMeth=Nearest
  Repeating Sequence : simulink/Sources/Repeating Sequence  rep_seq_t="[0  T/2 T]"  rep_seq_y=[0 1 0]
  VT1 : Outport  VectorParamsAs1DForOutWhenUnconnected=off
  VT2 : Outport  Port=2  VectorParamsAs1DForOutWhenUnconnected=off
  VT3 : Outport  Port=3  VectorParamsAs1DForOutWhenUnconnected=off
  VT4 : Outport  Port=4  VectorParamsAs1DForOutWhenUnconnected=off
  wires:
  Relational Operator/1 -> Product/1
  Repeating Sequence/1 -> Relational Operator4/2, Relational Operator/2
  In1/1 -> Relational Operator4/1, Relational Operator2/1, Relational Operator3/1, Relational Operator/1
  Constant/1 -> Relational Operator2/2, Relational Operator3/2
  Relational Operator3/1 -> Product/2
  Product/1 -> VT4/1, VT1/1
  Product3/1 -> VT3/1, VT2/1
  Relational Operator2/1 -> Product3/2
  Relational Operator4/1 -> Product3/1

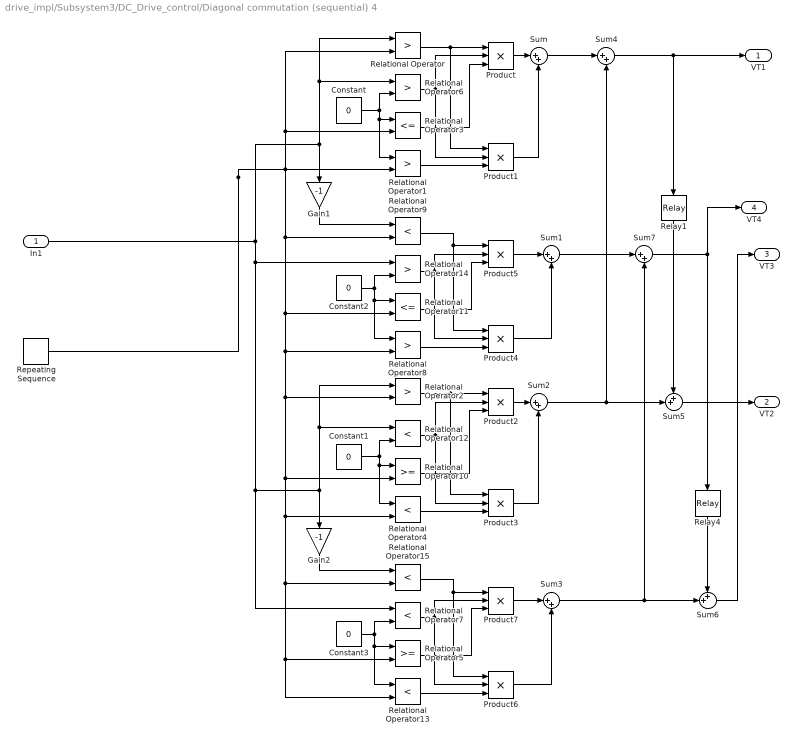
== system drive_impl/Subsystem3/DC_Drive_control/Diagonal commutation (sequential) 4 ==
  In1 : Inport
  Constant{,1..3} (4 alike) : Constant  Value=0
  Gain1 : Gain  Gain=-1
  Gain2 : Gain  Gain=-1
  Product{,1..7} (8 alike) : Product  Inputs=3
  Relational Operator{,1..2,6,8,14} (6 alike) : RelationalOperator  Operator=>  OutDataTypeStr=boolean  RndMeth=Nearest
  Relational Operator10 : RelationalOperator  OutDataTypeStr=boolean  RndMeth=Nearest
  Relational Operator11 : RelationalOperator  Operator=<=  OutDataTypeStr=boolean  RndMeth=Nearest
  Relational Operator{4,7,9,12..13,15} (6 alike) : RelationalOperator  Operator=<  OutDataTypeStr=boolean  RndMeth=Nearest
  Relational Operator3 : RelationalOperator  Operator=<=  OutDataTypeStr=boolean  RndMeth=Nearest
  Relational Operator5 : RelationalOperator  OutDataTypeStr=boolean  RndMeth=Nearest
  Relay1 : Relay  OnSwitchValue=0.999  OffSwitchValue=0.001  OnOutputValue=0  OffOutputValue=1
  Relay4 : Relay  OnSwitchValue=0.999  OffSwitchValue=0.001  OnOutputValue=0  OffOutputValue=1
  Repeating Sequence : simulink/Sources/Repeating Sequence  rep_seq_t="[0  T/2 T]"  rep_seq_y=[-1 1 -1]
  Sum{,1..4,7} (6 alike) : Sum  Inputs=|++
  Sum5 : Sum  Inputs=++|
  Sum6 : Sum  Inputs=++|
  VT1 : Outport  VectorParamsAs1DForOutWhenUnconnected=off
  VT2 : Outport  Port=2  VectorParamsAs1DForOutWhenUnconnected=off
  VT3 : Outport  Port=3  VectorParamsAs1DForOutWhenUnconnected=off
  VT4 : Outport  Port=4  VectorParamsAs1DForOutWhenUnconnected=off
  wires:
  Relational Operator10/1 -> Product2/3
  Relational Operator6/1 -> Product/2, Product1/2
  Relational Operator/1 -> Product/1, Product1/1
  Relational Operator3/1 -> Product/3
  Relational Operator9/1 -> Product5/1, Product4/1
  Product4/1 -> Sum1/2
  Constant2/1 -> Relational Operator11/1, Relational Operator8/1, Relational Operator14/2
  In1/1 -> Gain1/1, Relational Operator/1, Relational Operator6/1, Relational Operator14/1, Relational Operator7/1, Relational Operator12/1, Relational Operator2/1, Gain2/1
  Relational Operator14/1 -> Product5/2, Product4/2
  Product1/1 -> Sum/2
  Relational Operator1/1 -> Product1/3
  Constant/1 -> Relational Operator3/1, Relational Operator1/1, Relational Operator6/2
  Relay4/1 -> Sum6/1
  Relational Operator4/1 -> Product3/3
  Product/1 -> Sum/1
  Product5/1 -> Sum1/1
  Relational Operator8/1 -> Product4/3
  Product7/1 -> Sum3/1
  Repeating Sequence/1 -> Relational Operator1/2, Relational Operator/2, Relational Operator3/2, Relational Operator9/2, Relational Operator8/2, Relational Operator2/2, Relational Operator10/2, Relational Operator5/2, Relational Operator13/2, Relational Operator15/2, Relational Operator4/2, Relational Operator11/2
  Constant1/1 -> Relational Operator12/2, Relational Operator4/1, Relational Operator10/1
  Gain2/1 -> Relational Operator15/1
  Relational Operator5/1 -> Product7/3
  Relational Operator2/1 -> Product3/1, Product2/1
  Relational Operator11/1 -> Product5/3
  Sum1/1 -> Sum7/1
  Relational Operator12/1 -> Product3/2, Product2/2
  Relational Operator7/1 -> Product6/2, Product7/2
  Sum2/1 -> Sum5/2, Sum4/2
  Product2/1 -> Sum2/1
  Relational Operator13/1 -> Product6/3
  Sum/1 -> Sum4/1
  Sum4/1 -> VT1/1, Relay1/1
  Product6/1 -> Sum3/2
  Gain1/1 -> Relational Operator9/1
  Relational Operator15/1 -> Product6/1, Product7/1
  Constant3/1 -> Relational Operator7/2, Relational Operator13/1, Relational Operator5/1
  Product3/1 -> Sum2/2
  Sum7/1 -> Relay4/1, VT4/1
  Sum3/1 -> Sum6/2, Sum7/2
  Relay1/1 -> Sum5/1
  Sum5/1 -> VT2/1
  Sum6/1 -> VT3/1

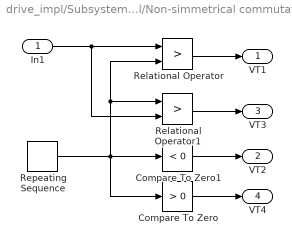
== system drive_impl/Subsystem3/DC_Drive_control/Non-simmetrical commutation 5 ==
  In1 : Inport
  Compare To Zero : simulink/Logic and Bit Operations/Compare To Zero  relop=>  OutDataTypeStr=boolean
  Compare To Zero1 : simulink/Logic and Bit Operations/Compare To Zero  relop=<  OutDataTypeStr=boolean
  Relational Operator : RelationalOperator  Operator=>  OutDataTypeStr=boolean  RndMeth=Nearest
  Relational Operator1 : RelationalOperator  Operator=>  OutDataTypeStr=boolean  RndMeth=Nearest
  Repeating Sequence : simulink/Sources/Repeating Sequence  rep_seq_t="[0  T ]"  rep_seq_y=[1 0]
  VT1 : Outport  VectorParamsAs1DForOutWhenUnconnected=off
  VT2 : Outport  Port=2  VectorParamsAs1DForOutWhenUnconnected=off
  VT3 : Outport  Port=3  VectorParamsAs1DForOutWhenUnconnected=off
  VT4 : Outport  Port=4  VectorParamsAs1DForOutWhenUnconnected=off
  wires:
  In1/1 -> Relational Operator/1, Relational Operator1/2
  Repeating Sequence/1 -> Compare To Zero/1, Relational Operator/2, Relational Operator1/1, Compare To Zero1/1
  Compare To Zero/1 -> VT4/1
  Relational Operator1/1 -> VT3/1
  Compare To Zero1/1 -> VT2/1
  Relational Operator/1 -> VT1/1

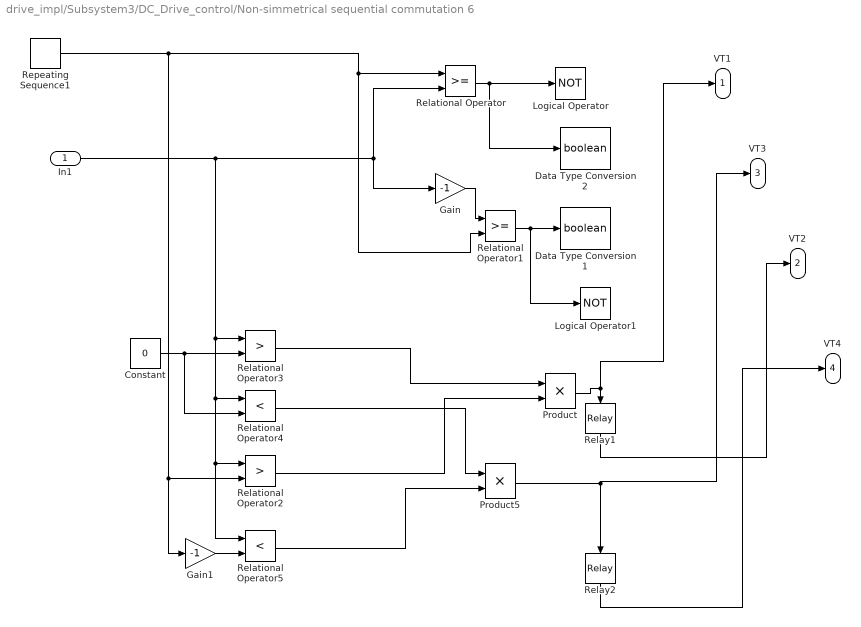
== system drive_impl/Subsystem3/DC_Drive_control/Non-simmetrical sequential commutation 6  ==
  In1 : Inport
  Constant : Constant  Value=0
  Data Type Conversion1 : DataTypeConversion  OutDataTypeStr=boolean  RndMeth=Ceiling  SaturateOnIntegerOverflow=on
  Data Type Conversion2 : DataTypeConversion  OutDataTypeStr=boolean  RndMeth=Ceiling  SaturateOnIntegerOverflow=on
  Gain : Gain  Gain=-1
  Gain1 : Gain  Gain=-1
  Logical Operator : Logic  Operator=NOT  AllPortsSameDT=off  OutDataTypeStr=boolean
  Logical Operator1 : Logic  Operator=NOT  AllPortsSameDT=off  OutDataTypeStr=boolean
  Product : Product
  Product5 : Product
  Relational Operator : RelationalOperator  OutDataTypeStr=boolean  RndMeth=Nearest
  Relational Operator1 : RelationalOperator  OutDataTypeStr=boolean  RndMeth=Nearest
  Relational Operator2 : RelationalOperator  Operator=>  OutDataTypeStr=boolean  RndMeth=Nearest
  Relational Operator3 : RelationalOperator  Operator=>  OutDataTypeStr=boolean  RndMeth=Nearest
  Relational Operator4 : RelationalOperator  Operator=<  OutDataTypeStr=boolean  RndMeth=Nearest
  Relational Operator5 : RelationalOperator  Operator=<  OutDataTypeStr=boolean  RndMeth=Nearest
  Relay1 : Relay  OnSwitchValue=0.9  OffSwitchValue=0.1  OnOutputValue=0  OffOutputValue=1
  Relay2 : Relay  OnSwitchValue=0.9  OffSwitchValue=0.1  OnOutputValue=0  OffOutputValue=1
  Repeating Sequence1 : simulink/Sources/Repeating Sequence  rep_seq_t="[0  T/2 T  ]"  rep_seq_y=[-1 1 -1]
  VT1 : Outport  VectorParamsAs1DForOutWhenUnconnected=off
  VT2 : Outport  Port=2  VectorParamsAs1DForOutWhenUnconnected=off
  VT3 : Outport  Port=3  VectorParamsAs1DForOutWhenUnconnected=off
  VT4 : Outport  Port=4  VectorParamsAs1DForOutWhenUnconnected=off
  wires:
  Gain/1 -> Relational Operator1/1
  Relational Operator/1 -> Logical Operator/1, Data Type Conversion2/1
  Relational Operator1/1 -> Logical Operator1/1, Data Type Conversion1/1
  Relay1/1 -> VT2/1
  In1/1 -> Relational Operator5/1, Relational Operator2/1, Relational Operator4/1, Relational Operator3/1, Gain/1, Relational Operator/2
  Product/1 -> VT1/1, Relay1/1
  Relational Operator3/1 -> Product/1
  Constant/1 -> Relational Operator4/2, Relational Operator3/2
  Gain1/1 -> Relational Operator5/2
  Product5/1 -> Relay2/1, VT3/1
  Relational Operator5/1 -> Product5/2
  Relational Operator4/1 -> Product5/1
  Repeating Sequence1/1 -> Gain1/1, Relational Operator2/2, Relational Operator/1, Relational Operator1/2
  Relational Operator2/1 -> Product/2
  Relay2/1 -> VT4/1

== system drive_impl/Subsystem3/DC_Drive_control/Symmetrical commutation 1 ==
  In1 : Inport
  Relational Operator : RelationalOperator  OutDataTypeStr=boolean  RndMeth=Nearest
  Relational Operator1 : RelationalOperator  Operator=<=  OutDataTypeStr=boolean  RndMeth=Nearest
  Repeating Sequence : simulink/Sources/Repeating Sequence  rep_seq_t="[0  T/2 T ]"  rep_seq_y=[0 0.99 0]
  VT1 : Outport  VectorParamsAs1DForOutWhenUnconnected=off
  VT2 : Outport  Port=2  VectorParamsAs1DForOutWhenUnconnected=off
  VT3 : Outport  Port=3  VectorParamsAs1DForOutWhenUnconnected=off
  VT4 : Outport  Port=4  VectorParamsAs1DForOutWhenUnconnected=off
  wires:
  Relational Operator1/1 -> VT2/1, VT3/1
  Repeating Sequence/1 -> Relational Operator/2, Relational Operator1/2
  In1/1 -> Relational Operator/1, Relational Operator1/1
  Relational Operator/1 -> VT1/1, VT4/1
